simulink model "ofur3"  (R2018b)
settings: Solver=VariableStepAuto  StartTime=0.0  StopTime=0.4  RelTol=1e-3
libraries: xbsIndex_r4 x31, commanapbnd3 x4
settings Model: Creator=IRZ  LastModifiedBy=IRZ

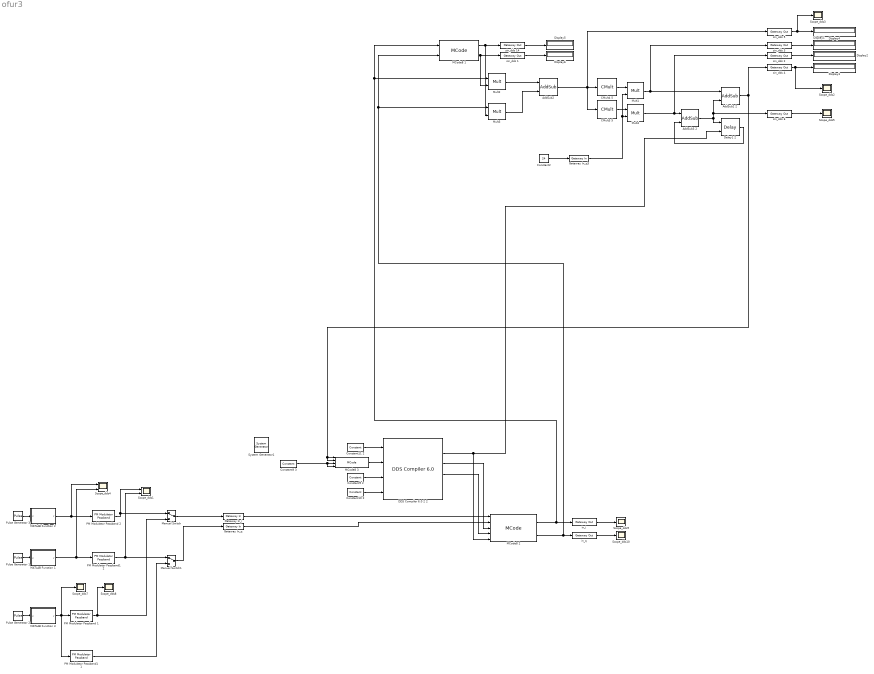
== system ofur3 ==
  " System Generator1" : xbsIndex_r4/ System Generator  Tag=genX  xilinxfamily=artix7  part=xc7a200t  speed=-3  package=fbg484  synthesis_tool=Vivado  clock_wrapper=Clock Enables  directory=C:/Users/IRZ/AppData/Roaming/Xilinx/Vivado/ofur_17  proj_type=Vivado  Synth_file=Vivado Synthesis Defaults  Impl_file=Vivado Implementation Defaults  testbench=off  simulink_period=1/30.72e6  sysclk_period=32.55  dcm_input_clock_period=10  incr_netlist=off  trim_vbits=Everywhere in SubSystem  dbl_ovrd=According to Block Masks  core_generation=According to Block Masks  run_coregen=off  deprecated_control=off  eval_field=0  block_type=sysgen
  AddSub2 : xbsIndex_r4/AddSub  mode=Subtraction  use_carryin=off  use_carryout=off  en=off  latency=1  precision=Full  arith_type=Unsigned  n_bits=16  bin_pt=14  quantization=Truncate  overflow=Wrap  use_behavioral_HDL=off  hw_selection=Fabric  pipelined=off  dbl_ovrd=off  block_type=addsub
  AddSub2 2 : xbsIndex_r4/AddSub  mode=Addition  use_carryin=off  use_carryout=off  en=off  latency=1  precision=User Defined  arith_type="Signed  (2's comp)"  n_bits=32  bin_pt=32  quantization=Truncate  overflow=Wrap  use_behavioral_HDL=off  hw_selection=Fabric  pipelined=off  dbl_ovrd=off  block_type=addsub
  AddSub3 2 : xbsIndex_r4/AddSub  mode=Addition  use_carryin=off  use_carryout=off  en=off  latency=0  precision=User Defined  arith_type="Signed  (2's comp)"  n_bits=48  bin_pt=48  quantization=Truncate  overflow=Wrap  use_behavioral_HDL=off  hw_selection=Fabric  pipelined=off  dbl_ovrd=off  block_type=addsub
  CMult3 5 : xbsIndex_r4/CMult  const=0.00000000010458116751  gui_display_data_type=Fixed-point  const_n_bits=48  const_bin_pt=48  float_type=Single  exp_bits=8  fraction_bits=24  en=off  latency=1  precision=User Defined  arith_type="Signed  (2's comp)"  n_bits=48  bin_pt=48  quantization=Truncate  overflow=Wrap  use_behavioral_HDL=off  mem_type=Distributed RAM  pipeline=off  dbl_ovrd=off  block_type=cmult
  CMult4 5 : xbsIndex_r4/CMult  const=0.0000102265908761675  gui_display_data_type=Fixed-point  const_n_bits=48  const_bin_pt=48  float_type=Single  exp_bits=8  fraction_bits=24  en=off  latency=1  precision=User Defined  arith_type="Signed  (2's comp)"  n_bits=48  bin_pt=48  quantization=Truncate  overflow=Wrap  use_behavioral_HDL=off  mem_type=Distributed RAM  pipeline=off  dbl_ovrd=off  block_type=cmult
  Constant10 2 : xbsIndex_r4/Constant  const=1.0  gui_display_data_type=Boolean  arith_type=Boolean  n_bits=16  bin_pt=14  preci_type=Single  exp_width=8  frac_width=24  explicit_period=on  period=1/30.72e6  equ=P=C  opselect=C  inp2=PCIN>>17  opr=+  inp1=P  carry=CIN  dbl_ovrd=off  block_type=constant
  Constant11 2 : xbsIndex_r4/Constant  const=1.0  gui_display_data_type=Boolean  arith_type=Boolean  n_bits=16  bin_pt=14  preci_type=Single  exp_width=8  frac_width=24  explicit_period=on  period=1/30.72e6  equ=P=C  opselect=C  inp2=PCIN>>17  opr=+  inp1=P  carry=CIN  dbl_ovrd=off  block_type=constant
  Constant2 : Constant  Value=24
  Constant9 2 : xbsIndex_r4/Constant  const=1.0  gui_display_data_type=Boolean  arith_type=Boolean  n_bits=16  bin_pt=14  preci_type=Single  exp_width=8  frac_width=24  explicit_period=on  period=1/30.72e6  equ=P=C  opselect=C  inp2=PCIN>>17  opr=+  inp1=P  carry=CIN  dbl_ovrd=off  block_type=constant
  Constant9 3 : xbsIndex_r4/Constant  const=0  gui_display_data_type=Fixed-point  arith_type=Unsigned  n_bits=32  bin_pt=32  preci_type=Single  exp_width=8  frac_width=24  explicit_period=on  period=1/30.72e6  equ=P=C  opselect=C  inp2=PCIN>>17  opr=+  inp1=P  carry=CIN  dbl_ovrd=off  block_type=constant
  DDS Compiler 6.0 2 2 : xbsIndex_r4/DDS Compiler 6.0   partspresent=Phase_Generator_and_SIN_COS_LUT  dds_clock_rate=30.72  channels=1  mode_of_operation=Standard  modulus=9  parameter_entry=Hardware_Parameters  spurious_free_dynamic_range=45  frequency_resolution=0.4  noise_shaping=None  phase_width=32  output_width=12  output_selection=Sine_and_Cosine  negative_sine=on  negative_cosine=on  amplitude_mode=Full_Range  memory_type=Auto  optimization_goal=Auto  dsp48_use=Minimal  resync=off  latency_configuration=Auto  latency=1  has_phase_out=on  has_aclken=off  has_aresetn=off  explicit_period=on  period=1/30.72e6  data_has_tlast=Not_Required  has_tready=on  s_phase_has_tuser=Not_Required  m_data_has_tuser=Not_Required  m_phase_has_tuser=Not_Required  s_phase_tuser_width=1  output_form=Twos_Complement  s_config_sync_mode=On_Vector  phase_increment=Streaming  output_frequency1=0  output_frequency2=0  output_frequency3=0  output_frequency4=0  output_frequency5=0  output_frequency6=0  output_frequency7=0  output_frequency8=0  output_frequency9=0  output_frequency10=0  output_frequency11=0  output_frequency12=0  output_frequency13=0  output_frequency14=0  output_frequency15=0  output_frequency16=0  pinc1='0'  pinc2='0'  pinc3='0'  pinc4='0'  pinc5='0'  pinc6='0'  pinc7='0'  pinc8='0'  pinc9='0'  pinc10='0'  pinc11='0'  pinc12='0'  pinc13='0'  pinc14='0'  pinc15='0'  pinc16='0'  phase_offset=Fixed  phase_offset_angles1=0  phase_offset_angles2=0  phase_offset_angles3=0  phase_offset_angles4=0  phase_offset_angles5=0  phase_offset_angles6=0  phase_offset_angles7=0  phase_offset_angles8=0  phase_offset_angles9=0  phase_offset_angles10=0  phase_offset_angles11=0  phase_offset_angles12=0  phase_offset_angles13=0  phase_offset_angles14=0  phase_offset_angles15=0  phase_offset_angles16=0  poff1='0'  poff2='0'  poff3='0'  poff4='0'  poff5='0'  poff6='0'  poff7='0'  poff8='0'  poff9='0'  poff10='0'  poff11='0'  poff12='0'  poff13='0'  poff14='0'  poff15='0'  poff16='0'  trim_axipin_name=on  simulation_type=hybrid_sim  simulation_model=sysgen:xddsv6_0_cmodel  data_path_portlist={ 's_axis_config_tdata_poff', 's_axis_config_tdata_chan0_poff', 's_axis_config_tdata_pinc', 's_axis_config_tdata_chan0_pinc', 's_axis_phase_tdata_resync', 's_axis_phase_tdata_chan0_resync', 's_axis_phase_tdata_poff', 's_axis_phase_tdata_chan0_poff', 's_axis_phase_tdata_pinc', 's_axis_phase_tdata_chan0_pinc', 's_axis_phase_tdata_phase_in', 'm_axis_data_tdata_sine', 'm_axis_data_tdata_chan0_sine', 'm_axis_data_tdata_cosine', 'm_axis_data_tdata_chan0_cosine', 'm_axis_phase_tdata_phase_out', 'm_axis_phase_tdata_chan0_phase_out'}  por_mode=false  gui_behaviour=Sysgen  ip_name=DDS Compiler  ip_version=6.0  dsptool_ready=true  wrapper_available=true  port_translation_map={ 'aclken' => 'en', 'aresetn' => 'rst' }  ipcore_usecache=true  ipcore_useipmodelcache=true  ipcore_xco_need_fpga_part=true  ipcore_verbose=false  block_type=dds_compiler_v6_0
  Delay1 2 : xbsIndex_r4/Delay  rst=off  infoeditControl=Selection of Reset will increase slice count due to use of real FFs and instead of SRLs  en=on  latency=1  reg_retiming=off  dbl_ovrd=off  block_type=delay
  Display{1..6} (6 alike) : Display
  Gateway In_i : xbsIndex_r4/Gateway In  gui_display_data_type=Fixed-point  arith_type="Signed  (2's comp)"  n_bits=12  bin_pt=11  preci_type=Single  exp_width=8  frac_width=24  rows=1  columns=1  quantization="Round  (unbiased: +/- Inf)"  overflow=Saturate  period=1/30720000  UseAsADC=off  ADCChannel='1'  interface=None  automatic_assignment=on  address_offset=hex2dec('00')  intf_name=''  intf_description=''  default_value=0  timing_constraint=None  locs_specified=off  LOCs={}  io_standard={}  inherit_from_input=off  hdl_port=on  dbl_ovrd=off  block_type=gatewayin
  Gateway In_q : xbsIndex_r4/Gateway In  gui_display_data_type=Fixed-point  arith_type="Signed  (2's comp)"  n_bits=12  bin_pt=11  preci_type=Single  exp_width=8  frac_width=24  rows=1  columns=1  quantization="Round  (unbiased: +/- Inf)"  overflow=Saturate  period=1/30720000  UseAsADC=off  ADCChannel='1'  interface=None  automatic_assignment=on  address_offset=hex2dec('00')  intf_name=''  intf_description=''  default_value=0  timing_constraint=None  locs_specified=off  LOCs={}  io_standard={}  inherit_from_input=off  hdl_port=on  dbl_ovrd=off  block_type=gatewayin
  Gateway In_q3 : xbsIndex_r4/Gateway In  gui_display_data_type=Fixed-point  arith_type="Signed  (2's comp)"  n_bits=10  bin_pt=0  preci_type=Single  exp_width=8  frac_width=24  rows=1  columns=1  quantization="Round  (unbiased: +/- Inf)"  overflow=Saturate  period=1/30720000  UseAsADC=off  ADCChannel='1'  interface=None  automatic_assignment=on  address_offset=hex2dec('00')  intf_name=''  intf_description=''  default_value=0  timing_constraint=None  locs_specified=off  LOCs={}  io_standard={}  inherit_from_input=off  hdl_port=on  dbl_ovrd=off  block_type=gatewayin
  MATLAB Function 1 : MATLAB Function  TreatAsAtomicUnit=on
  MATLAB Function 2 : MATLAB Function  TreatAsAtomicUnit=on
  MATLAB Function 3 : MATLAB Function  TreatAsAtomicUnit=on
  MCode8 1 : xbsIndex_r4/MCode  mfname=costas4  explicit_period=off  period=1/30.72e6  inputsTable={'boundInpExpr'=>['',''],'inputs'=>['im','qm']}  outputsTable={'outputs'=>['im_out','qm_out'],'suppressOut'=>['off','off']}  enable_stdout=off  enable_debug=off  suppress_output=on  defparams={}  hide_port_list={}  dbl_ovrd=off  block_type=mcode
  MCode8 2 : xbsIndex_r4/MCode  mfname=quadrature_detector  explicit_period=off  period=1/30.72e6  inputsTable={'boundInpExpr'=>['','','','',''],'inputs'=>['i','q','s','c','e']}  outputsTable={'outputs'=>['i_out','q_out'],'suppressOut'=>['off','off']}  enable_stdout=off  enable_debug=off  suppress_output=on  defparams={}  hide_port_list={}  dbl_ovrd=off  block_type=mcode
  MCode8 3 : xbsIndex_r4/MCode  mfname=dds_2  explicit_period=off  period=1/30.72e6  inputsTable={'boundInpExpr'=>['','','',''],'inputs'=>['looper','looper_min','furie','flag']}  outputsTable={'outputs'=>['z'],'suppressOut'=>['off']}  enable_stdout=off  enable_debug=off  suppress_output=on  defparams={}  hide_port_list={}  dbl_ovrd=off  block_type=mcode
  Manual Switch : ManualSwitch
  Manual Switch1 : ManualSwitch
  Mult1 : xbsIndex_r4/Mult  precision=User Defined  arith_type="Signed  (2's comp)"  n_bits=48  bin_pt=48  quantization=Truncate  overflow=Wrap  en=off  latency=1  use_behavioral_HDL=off  opt=Speed  use_embedded=on  optimum_pipeline=off  pipeline=on  dbl_ovrd=off  use_rpm=on  placement_style=Triangular  block_type=mult
  Mult2 : xbsIndex_r4/Mult  precision=Full  arith_type="Signed  (2's comp)"  n_bits=16  bin_pt=14  quantization=Truncate  overflow=Wrap  en=off  latency=0  use_behavioral_HDL=off  opt=Speed  use_embedded=on  optimum_pipeline=off  pipeline=on  dbl_ovrd=off  use_rpm=on  placement_style=Triangular  block_type=mult
  Mult3 : xbsIndex_r4/Mult  precision=Full  arith_type="Signed  (2's comp)"  n_bits=16  bin_pt=14  quantization=Truncate  overflow=Wrap  en=off  latency=0  use_behavioral_HDL=off  opt=Speed  use_embedded=on  optimum_pipeline=off  pipeline=on  dbl_ovrd=off  use_rpm=on  placement_style=Triangular  block_type=mult
  Mult4 : xbsIndex_r4/Mult  precision=User Defined  arith_type="Signed  (2's comp)"  n_bits=48  bin_pt=48  quantization=Truncate  overflow=Wrap  en=off  latency=1  use_behavioral_HDL=off  opt=Speed  use_embedded=on  optimum_pipeline=off  pipeline=on  dbl_ovrd=off  use_rpm=on  placement_style=Triangular  block_type=mult
  PM Modulator Passband 1 : commanapbnd3/PM Modulator Passband  Fc=1003000  Ph=0  Kc=pi/4
      settings: SourceProductName=Communications System Toolbox  SourceProductBaseCode=CM
  PM Modulator Passband 2 : commanapbnd3/PM Modulator Passband  Fc=1002000  Ph=0  Kc=pi/4
      settings: SourceProductName=Communications System Toolbox  SourceProductBaseCode=CM
  PM Modulator Passband1 1 : commanapbnd3/PM Modulator Passband  Fc=1003000  Ph=3*pi/2  Kc=pi/4
      settings: SourceProductName=Communications System Toolbox  SourceProductBaseCode=CM
  PM Modulator Passband1 2 : commanapbnd3/PM Modulator Passband  Fc=1002000  Ph=3*pi/2  Kc=pi/4
      settings: SourceProductName=Communications System Toolbox  SourceProductBaseCode=CM
  Pulse Generator 1 : DiscretePulseGenerator  Period=120  PulseWidth=60  PhaseDelay=60  SampleTime=1/30720000
  Pulse Generator 2 : DiscretePulseGenerator  Period=120  PulseWidth=60  SampleTime=1/30720000
  Pulse Generator 3 : DiscretePulseGenerator  Period=120  PulseWidth=60  SampleTime=1/30720000
  Scope_dds1 : Scope  NumInputPorts=2
  Scope_dds{2..3,5,7..10} (7 alike) : Scope
  Scope_dds4 : Scope  NumInputPorts=2
  in_i : xbsIndex_r4/Gateway Out  inherit_from_input=off  hdl_port=on  rows=1  columns=1  UseAsDAC=off  DACChannel='1'  interface=None  automatic_assignment=on  address_offset=hex2dec('00')  intf_name=''  intf_description=''  timing_constraint=None  locs_specified=off  LOCs={}  io_standard={}  block_type=gatewayout
  in_q : xbsIndex_r4/Gateway Out  inherit_from_input=off  hdl_port=on  rows=1  columns=1  UseAsDAC=off  DACChannel='1'  interface=None  automatic_assignment=on  address_offset=hex2dec('00')  intf_name=''  intf_description=''  timing_constraint=None  locs_specified=off  LOCs={}  io_standard={}  block_type=gatewayout
  sin_dds {1..6,14} (7 alike) : xbsIndex_r4/Gateway Out  inherit_from_input=off  hdl_port=off  rows=1  columns=1  UseAsDAC=off  DACChannel='1'  interface=None  automatic_assignment=on  address_offset=hex2dec('00')  intf_name=''  intf_description=''  timing_constraint=None  locs_specified=off  LOCs={}  io_standard={}  block_type=gatewayout
  wires:
  Mult4/1 -> sin_dds 2/1, AddSub3 2/1
  DDS Compiler 6.0 2 2/4 -> MCode8 2/4
  sin_dds 1/1 -> Display6/1
  Mult2/1 -> AddSub2/1
  MATLAB Function 1/1(y) -> PM Modulator Passband1 2/1, Scope_dds4/2
  PM Modulator Passband1 2/1 -> Scope_dds1/2, Manual Switch1/1
  MATLAB Function 2/1(y) -> PM Modulator Passband 2/1, Scope_dds4/1
  Constant9 2/1 -> DDS Compiler 6.0 2 2/3
  MCode8 1/1 -> Mult3/2, sin_dds 14/1
  Gateway In_q/1 -> MCode8 2/2
  DDS Compiler 6.0 2 2/3 -> MCode8 2/3
  Mult3/1 -> AddSub2/2
  PM Modulator Passband1 1/1 -> Manual Switch1/2
  AddSub2 2/1 -> MCode8 3/2, MCode8 3/1, sin_dds 4/1
  Manual Switch/1 -> Gateway In_i/1
  MATLAB Function 3/1(y) -> PM Modulator Passband 1/1, PM Modulator Passband1 1/1, Scope_dds7/1
  in_i/1 -> Scope_dds9/1
  MCode8 1/2 -> sin_dds 1/1, Mult2/2
  Gateway In_i/1 -> MCode8 2/1
  AddSub3 2/1 -> sin_dds 6/1, AddSub2 2/2, Delay1 2/1
  Constant11 2/1 -> DDS Compiler 6.0 2 2/1
  Pulse Generator 1/1 -> MATLAB Function 1/1(u)
  PM Modulator Passband 1/1 -> Scope_dds8/1, Manual Switch/2
  Manual Switch1/1 -> Gateway In_q/1
  Pulse Generator 2/1 -> MATLAB Function 3/1(u)
  MCode8 3/1 -> DDS Compiler 6.0 2 2/2
  sin_dds 14/1 -> Display5/1
  in_q/1 -> Scope_dds10/1
  Pulse Generator 3/1 -> MATLAB Function 2/1(u)
  Constant10 2/1 -> DDS Compiler 6.0 2 2/4
  Delay1 2/1 -> AddSub3 2/2
  PM Modulator Passband 2/1 -> Scope_dds1/1, Manual Switch/1
  sin_dds 2/1 -> Display2/1
  sin_dds 3/1 -> Display1/1
  sin_dds 4/1 -> Scope_dds2/1, Display3/1
  sin_dds 5/1 -> Scope_dds3/1, Display4/1
  sin_dds 6/1 -> Scope_dds5/1
  MCode8 2/2 -> Mult3/1, MCode8 1/2, in_q/1
  MCode8 2/1 -> Mult2/1, MCode8 1/1, in_i/1
  DDS Compiler 6.0 2 2/2 -> Delay1 2/2, MCode8 2/5
  AddSub2/1 -> CMult3 5/1, CMult4 5/1, sin_dds 5/1
  Constant9 3/1 -> MCode8 3/4, MCode8 3/3
  Constant2/1 -> Gateway In_q3/1
  Mult1/1 -> sin_dds 3/1, AddSub2 2/1
  CMult4 5/1 -> Mult1/1
  CMult3 5/1 -> Mult4/1
  Gateway In_q3/1 -> Mult1/2, Mult4/2

== matlab function ofur3/MATLAB Function 1 ==
  data: u input; y output
function y = fcn(u)

persistent B
persistent D
persistent E
persistent C
persistent F
persistent n

persistent A,

A = [1 7 7 1 7 3 5 5];
%A = [1 1 1 0 1 0 1 1 1 0 0 1 0 0 0 0];

%A = [0.707 0.707 0.707 0.707 0.707 -0.707 -0.707 -0.707];

if isempty(B)
 B = 0;
end

if isempty(D)
 D = 0;
end

if isempty(C)
 C = 0;
end

if isempty(F)
 F = 0;
end

if isempty(E)
 E = 0;
end

if isempty(n)
 n = 1;
end
 
D = B;
B = u;

if B == 0 && D == 1
    E = 1;
else
    E = 0;
end

if E == 1
    if n < 8
        n = n + 1;
    else
        n = 1;
    end
    C = A(n);

end

y = C;

== matlab function ofur3/MATLAB Function 3 ==
  data: u input; y output
function y = fcn(u)

persistent B
persistent D
persistent E
persistent C
persistent F
persistent n

persistent A,

A = [1 7 7 1 7 3 5 5];
%A = [1 1 1 0 1 0 1 1 1 0 0 1 0 0 0 0];

%A = [0.707 0.707 0.707 0.707 0.707 -0.707 -0.707 -0.707];

if isempty(B)
 B = 0;
end

if isempty(D)
 D = 0;
end

if isempty(C)
 C = 0;
end

if isempty(F)
 F = 0;
end

if isempty(E)
 E = 0;
end

if isempty(n)
 n = 1;
end
 
D = B;
B = u;

if B == 0 && D == 1
    E = 1;
else
    E = 0;
end

if E == 1
    if n < 8
        n = n + 1;
    else
        n = 1;
    end
    C = A(n);

end

y = C;

== matlab function ofur3/MATLAB Function 2 ==
  data: u input; y output
function y = fcn(u)

persistent B
persistent D
persistent E
persistent C
persistent F
persistent n

persistent A,

A = [1 7 7 1 7 3 5 5];
%A = [1 1 1 0 1 0 1 1 1 0 0 1 0 0 0 0];

%A = [0.707 0.707 0.707 0.707 0.707 -0.707 -0.707 -0.707];

if isempty(B)
 B = 0;
end

if isempty(D)
 D = 0;
end

if isempty(C)
 C = 0;
end

if isempty(F)
 F = 0;
end

if isempty(E)
 E = 0;
end

if isempty(n)
 n = 1;
end
 
D = B;
B = u;

if B == 0 && D == 1
    E = 1;
else
    E = 0;
end

if E == 1
    if n < 8
        n = n + 1;
    else
        n = 1;
    end
    C = A(n);

end

y = C;
